simulink model "Geneva_Drive"  (R2015a)
settings: Solver=ode15s  StartTime=0.0  StopTime=30  MaxStep=1e-2  RelTol=1e-4  AbsTol=1e-5
PostLoadFcn:
  | set_param(bdroot,'IgnoredZcDiagnostic','none')
  | warning off sm:compiler:topologyAnalysis:DanglingBlock
StartFcn:
  | tic;
StopFcn:
  | Elapsed_Sim_Time = toc;
  | disp(['Elapsed Sim Time = ' num2str(Elapsed_Sim_Time)]);
undefined symbols (not defined in the file): X, Y, Z
libraries: sm_lib x44, Contact_Forces_Lib x20, nesl_utility x5, simulink x1
(part 1 of 2)
Description:
  | Copyright 2015 The MathWorks, Inc.
settings Model: CovSFcnEnable=off  Creator=smiller  LastModifiedBy=smiller
settings DataIOCC: LimitDataPoints=off  SaveFormat=StructureWithTime  SaveState=on
settings DebuggingCC: IgnoredZcDiagnostic=none  SolverPrmCheckMsg=warning
settings ExplorerConfigSet: InternalSimMechanicsExplorerSettings="<ExplorerConfiguration><canonicalview>default</canonicalview><AnimationSetting><BasePlaybackSpeed>1.0</BasePlaybackSpeed><PlaybackSpeedFactor>4.0</PlaybackSpeedFactor></AnimationSetting><TilePanel><TileInfo><Tiles Columns=\"1\" Count=\"1\" Rows=\"1\"><Column Left=\"2\" Weight=\"1\"/><Column Left=\"677\"/><Row Top=\"2\" Weight=\"1\"/><Row Top=\"558\"/><Tile Height=\"1\" Width=\"1\" X=\"0\" Y=\"0\"/></Tiles></TileInfo><SceneInfo><SceneViewer><BGColor><R>0.93725490570068359</R><G>0.9686274528503418</G><B>0.9686274528503418</B></BGColor><Camera><Position><X>0.26080521668652706</X><Y>0.4639017710068058</Y><Z>0.36701914488687676</Z></Position><Center><X>-0.034093618327655228</X><Y>0.025639318022065816</Y><Z>-0.010275526182887462</Z></Center><Up><X>-0.45579088703273962</X><Y>0.73671340761661774</Y><Z>-0.4995077800553458</Z></Up><Left>-0.33774445205926895</Left><Right>0.33774445205926895</Right><Bottom>-0.208832748234272</Bottom><Top>0.208832748234272</Top></Camera></SceneViewer></SceneInfo></TilePanel></ExplorerConfiguration>"

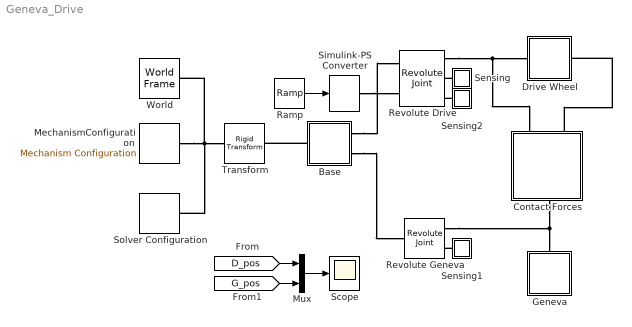
== system Geneva_Drive ==
  Base : Subsystem
  Contact Forces : Subsystem
  Drive Wheel : Subsystem
  Geneva : Subsystem
  MechanismConfiguration : sm_lib/Utilities/Mechanism Configuration  UniformGravity=Constant  GravityVector=[0 -9.81 0]  GravityUnits=m/s^2  LinearizationDelta=0.001  BlockFunction=simmechanics.library.utilities.mechanism_configuration
  Mux : Mux  Inputs=2
  Ramp : simulink/Sources/Ramp  slope=90  start=0  X0=106.26478005487978
  Revolute Drive : sm_lib/Joints/Revolute Joint  SenseConstraintForce=off  SenseConstraintForceX=off  SenseConstraintForceY=off  SenseConstraintForceZ=off  SenseConstraintTorque=off  SenseConstraintTorqueX=off  SenseConstraintTorqueY=off  SenseConstraintTorqueZ=off  SenseTotalForce=off  SenseTotalForceX=off  SenseTotalForceY=off  SenseTotalForceZ=off  SenseTotalTorque=off  SenseTotalTorqueX=off  SenseTotalTorqueY=off  SenseTotalTorqueZ=off  CompositeWrenchDir=FollowerOnBase  CompositeWrenchFrame=BaseFrame  EquilibriumPosition=0  EquilibriumPositionUnits=rad  SpringStiffness=0  SpringStiffnessUnits=m*N/rad  DampingCoefficient=0  DampingCoefficientUnits=m*s*N/rad  TorqueActuationMode=ComputedTorque  MotionActuationMode=InputMotion  SensePosition=on  SenseVelocity=off  SenseAcceleration=off  SenseTorqueForce=on  PositionTargetSpecify=on  PositionTargetPriority=Low  PositionTargetValue=106.26478005487978  PositionTargetValueUnits=deg  VelocityTargetSpecify=off  VelocityTargetPriority=High  VelocityTargetValue=0  VelocityTargetValueUnits=deg/s  BlockFunction=simmechanics.library.joints.revolute_joint
  Revolute Geneva : sm_lib/Joints/Revolute Joint  SenseConstraintForce=off  SenseConstraintForceX=off  SenseConstraintForceY=off  SenseConstraintForceZ=off  SenseConstraintTorque=off  SenseConstraintTorqueX=off  SenseConstraintTorqueY=off  SenseConstraintTorqueZ=off  SenseTotalForce=off  SenseTotalForceX=off  SenseTotalForceY=off  SenseTotalForceZ=off  SenseTotalTorque=off  SenseTotalTorqueX=off  SenseTotalTorqueY=off  SenseTotalTorqueZ=off  CompositeWrenchDir=FollowerOnBase  CompositeWrenchFrame=BaseFrame  EquilibriumPosition=90.000000000003197  EquilibriumPositionUnits=deg  SpringStiffness=0  SpringStiffnessUnits=m*N/rad  DampingCoefficient=1  DampingCoefficientUnits=m*s*N/rad  TorqueActuationMode=NoTorque  MotionActuationMode=ComputedMotion  SensePosition=on  SenseVelocity=off  SenseAcceleration=off  SenseTorqueForce=off  PositionTargetSpecify=on  PositionTargetPriority=Low  PositionTargetValue=90.000000000003197  PositionTargetValueUnits=deg  VelocityTargetSpecify=off  VelocityTargetPriority=High  VelocityTargetValue=0  VelocityTargetValueUnits=deg/s  BlockFunction=simmechanics.library.joints.revolute_joint
  Scope : Scope
      settings: YMin=0  YMax=8  SaveName=ScopeData3
  Sensing : Subsystem
  Sensing1 : Subsystem
  Sensing2 : Subsystem
  Simulink-PS Converter : nesl_utility/Simulink-PS Converter  PhysicalDomain=network_engine_domain  SubClassName=ps_input  LeftPortType=input  RightPortType=output  PseudoPeriodic=off  Frequencies=[]  NoiseDistribution=none  NoiseParameters=[]  Unit=deg  AffineConversion=off  InputFiltering=on  SimscapeFilterOrder=2  InputFilterTimeConstant=0.01  UdotUserProvided=1
  Solver Configuration : nesl_utility/Solver Configuration  PhysicalDomain=network_engine_domain  SubClassName=solver  LeftPortType=input  RightPortType=generic  Accelerate=off  Tones=[]  Harmonics=[]  SimulateNoise=off  Profile=off  UseLocalSampling=off  EnableSwitchedLinearOptims=on  FrequencyDomain=off  UseCCode=off  RelTol=0.001  AbsTol=1e-06  MinStep=1e-09  ToWorkspace=off  RevertToSquareIcSolve=off  NumHomotopyIterations=100  DoDC=off  ResidualTolerance=1e-09  UseLocalSolver=off  LocalSolverChoice=NE_BACKWARD_EULER_ADVANCER  LocalSolverSampleTime=0.001  DoFixedCost=off  MaxNonlinIter=3  MaxModeIter=2  LinearAlgebra=Sparse  DelaysMemoryBudget=1024  AutomaticFiltering=on  FilteringTimeConstant=0.001
  "Transform " : sm_lib/Frames and Transforms/Rigid Transform  TranslationMethod=Cartesian  TranslationLengthUnit=mm  TranslationStandardAxis=+Z  TranslationStandardOffset=0  TranslationCartesianOffset=[-30.994181557875464 40 -14.83110487348719]  TranslationROffset=0  TranslationROffsetUnits=m  TranslationZOffset=0  TranslationZOffsetUnits=m  TranslationThetaOffset=0  TranslationThetaOffsetUnits=deg  RotationMethod=ArbitraryAxis  RotationAngleUnits=rad  RotationStandardAxis=+Z  RotationAngle=1.5707963267948966  RotationArbitraryAxis=[-1 0 0]  FollAlignAxisA=+X  BaseAlignAxisA=+Y  FollAlignAxisB=+Y  BaseAlignAxisB=+Z  RotationMatrix=[1 0 0; 0 1 0; 0 0 1]  BlockFunction=simmechanics.library.frames_transforms.rigid_transform
  World : sm_lib/Frames and Transforms/World Frame  BlockFunction=simmechanics.library.frames_transforms.world_frame
  wires:
  Ramp/1 -> Simulink-PS Converter/1
  [D_pos] -> Mux/1
  Mux/1 -> Scope/1
  [G_pos] -> Mux/2
  connections:
  World/RConn1 -- "Transform "/LConn1 -- Solver Configuration/RConn1 -- MechanismConfiguration/RConn1
  Revolute Drive/RConn1 -- Drive Wheel/LConn1 -- Contact Forces/RConn1
  Revolute Geneva/RConn1 -- Geneva/LConn1 -- Contact Forces/LConn1
  Sensing2/LConn1 -- Revolute Drive/RConn3
  Sensing1/LConn1 -- Revolute Geneva/RConn2
  Sensing/LConn1 -- Revolute Drive/RConn2
  Contact Forces/RConn2 -- Drive Wheel/RConn1
  Simulink-PS Converter/RConn1 -- Revolute Drive/LConn2
  Base/LConn1 -- "Transform "/RConn1
  Base/RConn1 -- Revolute Drive/LConn1
  Base/RConn2 -- Revolute Geneva/LConn1

== system Geneva_Drive/Base ==
  ReferenceFrame : sm_lib/Frames and Transforms/Reference Frame  BlockFunction=simmechanics.library.frames_transforms.reference_frame
  Solid : sm_lib/Body Elements/Solid  InertiaType=Custom  Mass=5.6121441650895836  MassUnits=kg  CenterOfMass=[0.22415415704528135 0 -24.782168314450626]  CenterOfMassUnits=mm  MomentsOfInertia=[57246.923822174664 131168.16755878026 187513.90774897448]  MomentsOfInertiaUnits=kg*mm^2  ProductsOfInertia=[0 -24.879239071091789 0]  ProductsOfInertiaUnits=kg*mm^2  DensityBased=on  Density=1000  DensityUnits=kg/(m^3)  GraphicType=FromGeometry  MarkerShape=Sphere  MarkerSize=10  MarkerSizeUnits=m  GraphicVisPropType=SimpleVisualProperties  GraphicDiffuseColor=[0.82745098039215681 0.82745098039215681 0.81960784313725488]  GraphicSpecularColor=[0.5 0.5 0.5 1.0]  GraphicAmbientColor=[0.15 0.15 0.15 1.0]  GraphicEmissiveColor=[0.0 0.0 0.0 1.0]  GraphicShininess=75  GraphicOpacity=1  GeometryShape=FromFile  RectangleSize=[1 1]  RectangleSizeUnits=m  BrickDimensions=[1 1 1]  BrickDimensionUnits=m  CylinderRadius=1  CylinderRadiusUnits=m  CylinderLength=1  CylinderLengthUnits=m  SphereRadius=1  SphereRadiusUnits=m  EllipsoidRadii=[1 1 1]  EllipsoidRadiiUnits=m  ExtrusionCrossSection=[1 1; -1 1; -1 -1; 1 -1]  ExtrusionCrossSectionUnits=m  ExtrusionLength=1  ExtrusionLengthUnits=m  PolygonNumSides=3  PolygonOuterRadius=1  PolygonOuterRadiusUnits=m  ExtGeomFileType=STL  ExtGeomFileName=Base_Default_sldprt.STL  ExtGeomFileUnits=mm  RevolutionCrossSection=[1 1; 1 -1; 2 -1; 2 1]  RevolutionCrossSectionUnits=m  RevolutionExtent=Full  RevolutionAngle=180  RevolutionAngleUnits=deg  BlockFunction=simmechanics.library.body_elements.solid
  Transform : sm_lib/Frames and Transforms/Rigid Transform  TranslationMethod=Cartesian  TranslationLengthUnit=mm  TranslationStandardAxis=+Z  TranslationStandardOffset=0  TranslationCartesianOffset=[100 0 0]  TranslationROffset=0  TranslationROffsetUnits=m  TranslationZOffset=0  TranslationZOffsetUnits=m  TranslationThetaOffset=0  TranslationThetaOffsetUnits=deg  RotationMethod=ArbitraryAxis  RotationAngleUnits=rad  RotationStandardAxis=+Z  RotationAngle=0  RotationArbitraryAxis=[0 0 0]  FollAlignAxisA=+X  BaseAlignAxisA=+Y  FollAlignAxisB=+Y  BaseAlignAxisB=+Z  RotationMatrix=[1 0 0; 0 1 0; 0 0 1]  BlockFunction=simmechanics.library.frames_transforms.rigid_transform
  Transform2 : sm_lib/Frames and Transforms/Rigid Transform  TranslationMethod=Cartesian  TranslationLengthUnit=mm  TranslationStandardAxis=+Z  TranslationStandardOffset=0  TranslationCartesianOffset=[-99.999999999999986 0 57.42640687119286]  TranslationROffset=0  TranslationROffsetUnits=m  TranslationZOffset=0  TranslationZOffsetUnits=m  TranslationThetaOffset=0  TranslationThetaOffsetUnits=deg  RotationMethod=ArbitraryAxis  RotationAngleUnits=rad  RotationStandardAxis=+Z  RotationAngle=3.1415926535897931  RotationArbitraryAxis=[1 0 0]  FollAlignAxisA=+X  BaseAlignAxisA=+Y  FollAlignAxisB=+Y  BaseAlignAxisB=+Z  RotationMatrix=[1 0 0; 0 1 0; 0 0 1]  BlockFunction=simmechanics.library.frames_transforms.rigid_transform
  F3 : PMIOPort  Port=1  Side=Left
  F2 : PMIOPort  Port=2  Side=Right
  F : PMIOPort  Port=3  Side=Right
  connections:
  Transform2/RConn1 -- F2/RConn1
  Transform/RConn1 -- F/RConn1
  F3/RConn1 -- Transform2/LConn1 -- Transform/LConn1 -- ReferenceFrame/RConn1 -- Solid/RConn1

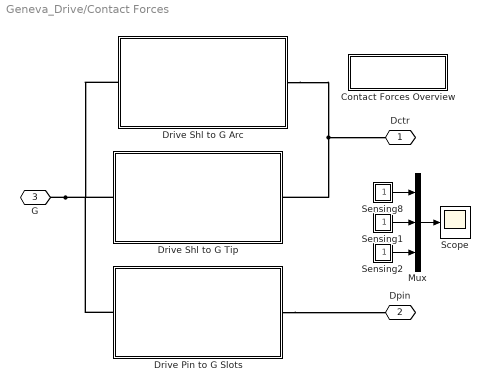
== system Geneva_Drive/Contact Forces ==
  Contact Forces Overview : Subsystem
      settings: OpenFcn=web(which('Geneva_Drive_Contact_Forces.html'));
      mask Display: disp('Contact Forces\nOverview');
  Drive Pin to G Slots : Subsystem  mask(Contact Forces, Drive Pin and Geneva Slot){k_contact=1e5, b_contact=1e4, r_drive_pin=0.015, d_genv_lin=0.0055, l_genv_lin=0.1405*2}
      mask prompts: k_contact "Contact Stiffness (N/m)"; b_contact "Contact Damping (N/(m/s))"; r_drive_pin "Radius of Drive Wheel Pin (m)"; d_genv_lin "Line Thickness, Geneva Slot Contact (m)"; l_genv_lin "Slot Length Through Geneva (m)"
      mask help:
      | This subsystem models the contact forces between the drive wheel pin and the four slots on the Geneva.  All contact forces are identical.  They connect one reference frame on the drive wheel pin and four reference frames on the Geneva.
      |
      | Click the Help button for a diagram of the contact forces and the parameters.
      mask Help: web(which('Geneva_Drive_Contact_DPin_GSlot.html'));
      mask Display:
      | image(imread('Contact_Diagram_Dpin_to_GSlot_IMAGE.jpg'));
      | port_label('LConn',1,'LinB');
      | port_label('RConn',1,'CirF');
  Drive Shl to G Arc : Subsystem  mask(Contact Forces, Drive Shoulder and Geneva Arc){k_contact=1e4, b_contact=1e2, r_shld_cir=0.005, r_genv_xcir=0.115, d_genv_xcir=0.005, d_genv_ctr_to_xcir=0.2}
      mask prompts: k_contact "Contact Stiffness (N/m)"; b_contact "Contact Damping (N/(m/s))"; r_shld_cir "Circle Radius of Drive Wheel Shoulder Contact (m)"; r_genv_xcir "Ring Radius, Geneva Arc (m)"; d_genv_xcir "Ring Thickness, Geneva Arc Contact (m)"; d_genv_ctr_to_xcir "Distance Geneva axis to center exterior circle (m)"
      mask help:
      | This subsystem models the contact forces between the drive wheel shoulder and the exterior arcs on the Geneva.  All contact forces are identical.  They connect two reference frames on the drive wheel and four reference frames on the Geneva.
      |
      | Click the Help button for a diagram of the contact forces and the parameters.
      mask Help: web(which('Geneva_Drive_Contact_Shld_Garc.html'));
      mask Display:
      | image(imread('Contact_Diagram_Shld_to_GArc_IMAGE.jpg'));
      | port_label('Lconn',1,'RinB');
      | port_label('Rconn',1,'CirF');
  Drive Shl to G Tip : Subsystem  mask(Contact Forces, Drive Shoulder and Geneva Tips){k_contact=1e4, b_contact=1e2, r_genv_cir=0.0045, r_shld=0.115, d_shld=0.005}
      mask prompts: k_contact "Contact Stiffness (N/m)"; b_contact "Contact Damping (N/(m/s))"; r_genv_cir "Circle Radius, Geneva Tip Contact (m)"; r_shld "Ring Radius, Drive Wheel Shoulder (m)"; d_shld "Ring Thickness, Drive Wheel Shoulder Contact (m)"
      mask help:
      | This subsystem models the contact forces between the drive wheel shoulder and the tips of the Geneva.  All contact forces are identical.  They connect one reference frame on the drive wheel and eight reference frames on the Geneva.
      |
      | Click the Help button for a diagram of the contact forces and the parameters.
      mask Help: web(which('Geneva_Drive_Contact_Shld_Gtip.html'));
      mask Display:
      | image(imread('Contact_Diagram_Gtip_to_Shld_IMAGE.jpg'));
      | port_label('Lconn',1,'CirF');
      | port_label('Rconn',1,'RinB');
  Mux : Mux  Inputs=3
  Scope : Scope
      settings: YMin=-10  YMax=60  SaveName=ScopeData5
  Sensing1 : Subsystem
  Sensing2 : Subsystem
  Sensing8 : Subsystem
  Dctr : PMIOPort  Port=1  Side=Right
  Dpin : PMIOPort  Port=2  Side=Right
  G : PMIOPort  Port=3  Side=Left
  wires:
  Mux/1 -> Scope/1
  Sensing2/1(S) -> Mux/3
  Sensing1/1(S) -> Mux/2
  Sensing8/1(S) -> Mux/1
  connections:
  G/RConn1 -- Drive Shl to G Arc/LConn1 -- Drive Pin to G Slots/LConn1 -- Drive Shl to G Tip/LConn1
  Drive Pin to G Slots/RConn1 -- Dpin/RConn1
  Drive Shl to G Arc/RConn1 -- Dctr/RConn1 -- Drive Shl to G Tip/RConn1

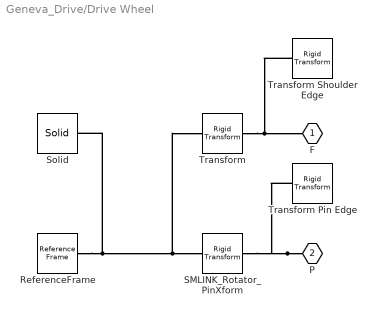
== system Geneva_Drive/Drive Wheel ==
  ReferenceFrame : sm_lib/Frames and Transforms/Reference Frame  BlockFunction=simmechanics.library.frames_transforms.reference_frame
  SMLINK_Rotator_PinXform : sm_lib/Frames and Transforms/Rigid Transform  TranslationMethod=Cartesian  TranslationLengthUnit=mm  TranslationStandardAxis=+Z  TranslationStandardOffset=0  TranslationCartesianOffset=[0 99.999999999999943 1.0000000000000009]  TranslationROffset=0  TranslationROffsetUnits=m  TranslationZOffset=0  TranslationZOffsetUnits=m  TranslationThetaOffset=0  TranslationThetaOffsetUnits=deg  RotationMethod=StandardAxis  RotationAngleUnits=deg  RotationStandardAxis=+Z  RotationAngle=10  RotationArbitraryAxis=[0 0 1]  FollAlignAxisA=+X  BaseAlignAxisA=+Y  FollAlignAxisB=+Y  BaseAlignAxisB=+Z  RotationMatrix=[1 0 0; 0 1 0; 0 0 1]  BlockFunction=simmechanics.library.frames_transforms.rigid_transform
  Solid : sm_lib/Body Elements/Solid  InertiaType=Custom  Mass=1.1459440199505517  MassUnits=kg  CenterOfMass=[-103.32572655678197 -3.3257265567819814 0.56035000006051983]  CenterOfMassUnits=mm  MomentsOfInertia=[5063.1142307875289 5063.1142307875298 10008.151794093599]  MomentsOfInertiaUnits=kg*mm^2  ProductsOfInertia=[46.956086417341879 46.956086417341901 41.94861289102812]  ProductsOfInertiaUnits=kg*mm^2  DensityBased=on  Density=1000  DensityUnits=kg/(m^3)  GraphicType=FromGeometry  MarkerShape=Sphere  MarkerSize=10  MarkerSizeUnits=m  GraphicVisPropType=SimpleVisualProperties  GraphicDiffuseColor=[0.2 0.4 1.0]  GraphicSpecularColor=[0.5 0.5 0.5 1.0]  GraphicAmbientColor=[0.15 0.15 0.15 1.0]  GraphicEmissiveColor=[0.0 0.0 0.0 1.0]  GraphicShininess=75  GraphicOpacity=1  GeometryShape=FromFile  RectangleSize=[1 1]  RectangleSizeUnits=m  BrickDimensions=[1 1 1]  BrickDimensionUnits=m  CylinderRadius=1  CylinderRadiusUnits=m  CylinderLength=1  CylinderLengthUnits=m  SphereRadius=1  SphereRadiusUnits=m  EllipsoidRadii=[1 1 1]  EllipsoidRadiiUnits=m  ExtrusionCrossSection=[1 1; -1 1; -1 -1; 1 -1]  ExtrusionCrossSectionUnits=m  ExtrusionLength=1  ExtrusionLengthUnits=m  PolygonNumSides=3  PolygonOuterRadius=1  PolygonOuterRadiusUnits=m  ExtGeomFileType=STL  ExtGeomFileName=Drive_Wheel_Default_sldprt.STL  ExtGeomFileUnits=mm  RevolutionCrossSection=[1 1; 1 -1; 2 -1; 2 1]  RevolutionCrossSectionUnits=m  RevolutionExtent=Full  RevolutionAngle=180  RevolutionAngleUnits=deg  BlockFunction=simmechanics.library.body_elements.solid
  Transform : sm_lib/Frames and Transforms/Rigid Transform  TranslationMethod=Cartesian  TranslationLengthUnit=mm  TranslationStandardAxis=+Z  TranslationStandardOffset=0  TranslationCartesianOffset=[-100.00000000000026 2.1316282072803006e-14 57.426406871192782]  TranslationROffset=0  TranslationROffsetUnits=m  TranslationZOffset=0  TranslationZOffsetUnits=m  TranslationThetaOffset=0  TranslationThetaOffsetUnits=deg  RotationMethod=ArbitraryAxis  RotationAngleUnits=rad  RotationStandardAxis=+Z  RotationAngle=3.1415926535897931  RotationArbitraryAxis=[-1 5.9163189700902024e-33 -6.6609835156154749e-17]  FollAlignAxisA=+X  BaseAlignAxisA=+Y  FollAlignAxisB=+Y  BaseAlignAxisB=+Z  RotationMatrix=[1 0 0; 0 1 0; 0 0 1]  BlockFunction=simmechanics.library.frames_transforms.rigid_transform
  Transform Pin Edge : sm_lib/Frames and Transforms/Rigid Transform  TranslationMethod=StandardAxis  TranslationLengthUnit=m  TranslationStandardAxis=+X  TranslationStandardOffset=0.015  TranslationCartesianOffset=[0 0 0]  TranslationROffset=0.115  TranslationROffsetUnits=m  TranslationZOffset=0  TranslationZOffsetUnits=m  TranslationThetaOffset=270  TranslationThetaOffsetUnits=deg  RotationMethod=None  RotationAngleUnits=deg  RotationStandardAxis=+Z  RotationAngle=0  RotationArbitraryAxis=[0 0 1]  FollAlignAxisA=+X  BaseAlignAxisA=+Y  FollAlignAxisB=+Y  BaseAlignAxisB=+Z  RotationMatrix=[1 0 0; 0 1 0; 0 0 1]  BlockFunction=simmechanics.library.frames_transforms.rigid_transform
  Transform Shoulder Edge : sm_lib/Frames and Transforms/Rigid Transform  TranslationMethod=Cylindrical  TranslationLengthUnit=m  TranslationStandardAxis=+X  TranslationStandardOffset=0.115  TranslationCartesianOffset=[0 0 0]  TranslationROffset=0.115  TranslationROffsetUnits=m  TranslationZOffset=0  TranslationZOffsetUnits=m  TranslationThetaOffset=270  TranslationThetaOffsetUnits=deg  RotationMethod=None  RotationAngleUnits=deg  RotationStandardAxis=+Z  RotationAngle=0  RotationArbitraryAxis=[0 0 1]  FollAlignAxisA=+X  BaseAlignAxisA=+Y  FollAlignAxisB=+Y  BaseAlignAxisB=+Z  RotationMatrix=[1 0 0; 0 1 0; 0 0 1]  BlockFunction=simmechanics.library.frames_transforms.rigid_transform
  F : PMIOPort  Port=1  Side=Left
  P : PMIOPort  Port=2  Side=Right
  connections:
  Transform Shoulder Edge/LConn1 -- F/RConn1 -- Transform/RConn1
  P/RConn1 -- Transform Pin Edge/LConn1 -- SMLINK_Rotator_PinXform/RConn1
  ReferenceFrame/RConn1 -- Solid/RConn1 -- Transform/LConn1 -- SMLINK_Rotator_PinXform/LConn1

== system Geneva_Drive/Geneva ==
  ReferenceFrame : sm_lib/Frames and Transforms/Reference Frame  BlockFunction=simmechanics.library.frames_transforms.reference_frame
  Solid : sm_lib/Body Elements/Solid  InertiaType=Custom  Mass=0.24105441419713447  MassUnits=kg  CenterOfMass=[100.00000000000023 1.1564451014440063e-12 5.0000000000000009]  CenterOfMassUnits=mm  MomentsOfInertia=[803.62795532691052 803.62795532691234 1603.261580672231]  MomentsOfInertiaUnits=kg*mm^2  ProductsOfInertia=[0 0 0]  ProductsOfInertiaUnits=kg*mm^2  DensityBased=on  Density=1000  DensityUnits=kg/(m^3)  GraphicType=FromGeometry  MarkerShape=Sphere  MarkerSize=10  MarkerSizeUnits=m  GraphicVisPropType=SimpleVisualProperties  GraphicDiffuseColor=[1.0 0.4 0.0]  GraphicSpecularColor=[0.5 0.5 0.5 1.0]  GraphicAmbientColor=[0.15 0.15 0.15 1.0]  GraphicEmissiveColor=[0.0 0.0 0.0 1.0]  GraphicShininess=75  GraphicOpacity=1  GeometryShape=FromFile  RectangleSize=[1 1]  RectangleSizeUnits=m  BrickDimensions=[1 1 1]  BrickDimensionUnits=m  CylinderRadius=1  CylinderRadiusUnits=m  CylinderLength=1  CylinderLengthUnits=m  SphereRadius=1  SphereRadiusUnits=m  EllipsoidRadii=[1 1 1]  EllipsoidRadiiUnits=m  ExtrusionCrossSection=[1 1; -1 1; -1 -1; 1 -1]  ExtrusionCrossSectionUnits=m  ExtrusionLength=1  ExtrusionLengthUnits=m  PolygonNumSides=3  PolygonOuterRadius=1  PolygonOuterRadiusUnits=m  ExtGeomFileType=STL  ExtGeomFileName=Geneva_Default_sldprt.STL  ExtGeomFileUnits=mm  RevolutionCrossSection=[1 1; 1 -1; 2 -1; 2 1]  RevolutionCrossSectionUnits=m  RevolutionExtent=Full  RevolutionAngle=180  RevolutionAngleUnits=deg  BlockFunction=simmechanics.library.body_elements.solid
  Transform Ref to Ctr : sm_lib/Frames and Transforms/Rigid Transform  TranslationMethod=Cartesian  TranslationLengthUnit=mm  TranslationStandardAxis=+Z  TranslationStandardOffset=0  TranslationCartesianOffset=[99.999999999999261 -2.4158453015843406e-13 -1.4210854715202004e-14]  TranslationROffset=0  TranslationROffsetUnits=m  TranslationZOffset=0  TranslationZOffsetUnits=m  TranslationThetaOffset=0  TranslationThetaOffsetUnits=deg  RotationMethod=ArbitraryAxis  RotationAngleUnits=rad  RotationStandardAxis=+Z  RotationAngle=0  RotationArbitraryAxis=[0 0 0]  FollAlignAxisA=+X  BaseAlignAxisA=+Y  FollAlignAxisB=+Y  BaseAlignAxisB=+Z  RotationMatrix=[1 0 0; 0 1 0; 0 0 1]  BlockFunction=simmechanics.library.frames_transforms.rigid_transform
  F : PMIOPort  Port=1  Side=Left
  connections:
  F/RConn1 -- Transform Ref to Ctr/RConn1
  Transform Ref to Ctr/LConn1 -- ReferenceFrame/RConn1 -- Solid/RConn1

== system Geneva_Drive/Sensing ==
  PS-Simulink Converter : nesl_utility/PS-Simulink Converter  PhysicalDomain=network_engine_domain  SubClassName=ps_output  LeftPortType=input  RightPortType=output  PseudoPeriodic=off  Frequencies=[]  Unit=rev  AffineConversion=off
  S : PMIOPort  Port=1  Side=Left
  tag scope: D_pos=global
  wires:
  PS-Simulink Converter/1 -> [D_pos]
  connections:
  PS-Simulink Converter/LConn1 -- S/RConn1

== system Geneva_Drive/Sensing1 ==
  PS-Simulink Converter : nesl_utility/PS-Simulink Converter  PhysicalDomain=network_engine_domain  SubClassName=ps_output  LeftPortType=input  RightPortType=output  PseudoPeriodic=off  Frequencies=[]  Unit=rev  AffineConversion=off
  S : PMIOPort  Port=1  Side=Left
  tag scope: G_pos=global
  wires:
  PS-Simulink Converter/1 -> [G_pos]
  connections:
  PS-Simulink Converter/LConn1 -- S/RConn1

== system Geneva_Drive/Sensing2 ==
  PS-Simulink Converter : nesl_utility/PS-Simulink Converter  PhysicalDomain=network_engine_domain  SubClassName=ps_output  LeftPortType=input  RightPortType=output  PseudoPeriodic=off  Frequencies=[]  Unit=1  AffineConversion=off
  Scope : Scope
  S : PMIOPort  Port=1  Side=Left
  wires:
  PS-Simulink Converter/1 -> Scope/1
  connections:
  PS-Simulink Converter/LConn1 -- S/RConn1

== system Geneva_Drive/Contact Forces/Contact Forces Overview ==

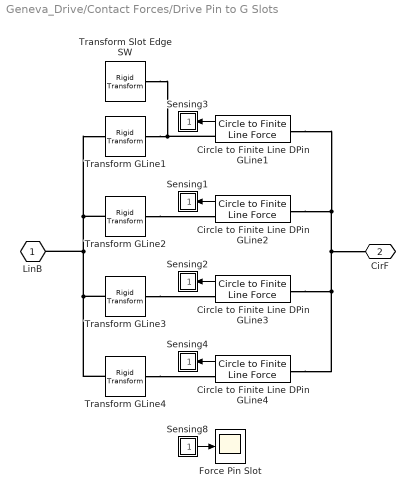
== system Geneva_Drive/Contact Forces/Drive Pin to G Slots ==
  Circle to Finite Line DPin GLine{1..4} (4 alike) : Contact_Forces_Lib/2D/Circle to Finite Line Force  circle_rad=r_drive_pin  line_depth=d_genv_lin  line_length=l_genv_lin  force_law=Linear  k_contact=k_contact  b_contact=b_contact  pen_full_damp_F=1e-4  pen_exponent=1  custom_param_1=1  custom_param_2=1  friction_law=None  mu_kinetic=0.5  mu_static=0.7  v_thr=0.001
  Force Pin Slot : Scope
      settings: YMin=0  YMax=60
  Sensing1 : Subsystem
  Sensing2 : Subsystem
  Sensing3 : Subsystem
  Sensing4 : Subsystem
  Sensing8 : Subsystem
  Transform GLine1 : sm_lib/Frames and Transforms/Rigid Transform  TranslationMethod=Cylindrical  TranslationLengthUnit=m  TranslationStandardAxis=+Z  TranslationStandardOffset=0  TranslationCartesianOffset=[0 0 0]  TranslationROffset=-0.02  TranslationROffsetUnits=m  TranslationZOffset=0  TranslationZOffsetUnits=m  TranslationThetaOffset=315  TranslationThetaOffsetUnits=deg  RotationMethod=StandardAxis  RotationAngleUnits=deg  RotationStandardAxis=+Z  RotationAngle=315  RotationArbitraryAxis=[0 0 1]  FollAlignAxisA=+X  BaseAlignAxisA=+Y  FollAlignAxisB=+Y  BaseAlignAxisB=+Z  RotationMatrix=[1 0 0; 0 1 0; 0 0 1]  BlockFunction=simmechanics.library.frames_transforms.rigid_transform
  Transform GLine2 : sm_lib/Frames and Transforms/Rigid Transform  TranslationMethod=Cylindrical  TranslationLengthUnit=m  TranslationStandardAxis=+Z  TranslationStandardOffset=0  TranslationCartesianOffset=[0 0 0]  TranslationROffset=-0.02  TranslationROffsetUnits=m  TranslationZOffset=0  TranslationZOffsetUnits=m  TranslationThetaOffset=135  TranslationThetaOffsetUnits=deg  RotationMethod=StandardAxis  RotationAngleUnits=deg  RotationStandardAxis=+Z  RotationAngle=135  RotationArbitraryAxis=[0 0 1]  FollAlignAxisA=+X  BaseAlignAxisA=+Y  FollAlignAxisB=+Y  BaseAlignAxisB=+Z  RotationMatrix=[1 0 0; 0 1 0; 0 0 1]  BlockFunction=simmechanics.library.frames_transforms.rigid_transform
  Transform GLine3 : sm_lib/Frames and Transforms/Rigid Transform  TranslationMethod=Cylindrical  TranslationLengthUnit=m  TranslationStandardAxis=+Z  TranslationStandardOffset=0  TranslationCartesianOffset=[0 0 0]  TranslationROffset=-0.02  TranslationROffsetUnits=m  TranslationZOffset=0  TranslationZOffsetUnits=m  TranslationThetaOffset=225  TranslationThetaOffsetUnits=deg  RotationMethod=StandardAxis  RotationAngleUnits=deg  RotationStandardAxis=+Z  RotationAngle=225  RotationArbitraryAxis=[0 0 1]  FollAlignAxisA=+X  BaseAlignAxisA=+Y  FollAlignAxisB=+Y  BaseAlignAxisB=+Z  RotationMatrix=[1 0 0; 0 1 0; 0 0 1]  BlockFunction=simmechanics.library.frames_transforms.rigid_transform
  Transform GLine4 : sm_lib/Frames and Transforms/Rigid Transform  TranslationMethod=Cylindrical  TranslationLengthUnit=m  TranslationStandardAxis=+Z  TranslationStandardOffset=0  TranslationCartesianOffset=[0 0 0]  TranslationROffset=-0.02  TranslationROffsetUnits=m  TranslationZOffset=0  TranslationZOffsetUnits=m  TranslationThetaOffset=45  TranslationThetaOffsetUnits=deg  RotationMethod=StandardAxis  RotationAngleUnits=deg  RotationStandardAxis=+Z  RotationAngle=45  RotationArbitraryAxis=[0 0 1]  FollAlignAxisA=+X  BaseAlignAxisA=+Y  FollAlignAxisB=+Y  BaseAlignAxisB=+Z  RotationMatrix=[1 0 0; 0 1 0; 0 0 1]  BlockFunction=simmechanics.library.frames_transforms.rigid_transform
  Transform Slot Edge SW : sm_lib/Frames and Transforms/Rigid Transform  TranslationMethod=StandardAxis  TranslationLengthUnit=m  TranslationStandardAxis=+X  TranslationStandardOffset=0.005  TranslationCartesianOffset=[0 0 0]  TranslationROffset=0  TranslationROffsetUnits=m  TranslationZOffset=0  TranslationZOffsetUnits=m  TranslationThetaOffset=0  TranslationThetaOffsetUnits=deg  RotationMethod=None  RotationAngleUnits=deg  RotationStandardAxis=+Z  RotationAngle=45  RotationArbitraryAxis=[0 0 1]  FollAlignAxisA=+X  BaseAlignAxisA=+Y  FollAlignAxisB=+Y  BaseAlignAxisB=+Z  RotationMatrix=[1 0 0; 0 1 0; 0 0 1]  BlockFunction=simmechanics.library.frames_transforms.rigid_transform
  LinB : PMIOPort  Port=1  Side=Left
  CirF : PMIOPort  Port=2  Side=Right
  wires:
  Sensing8/1(S) -> Force Pin Slot/1
  Circle to Finite Line DPin GLine4/1 -> Sensing4/1(S)
  Circle to Finite Line DPin GLine3/1 -> Sensing2/1(S)
  Circle to Finite Line DPin GLine2/1 -> Sensing1/1(S)
  Circle to Finite Line DPin GLine1/1 -> Sensing3/1(S)
  connections:
  Transform GLine2/RConn1 -- Circle to Finite Line DPin GLine2/RConn1
  Transform GLine3/RConn1 -- Circle to Finite Line DPin GLine3/RConn1
  Circle to Finite Line DPin GLine4/LConn1 -- CirF/RConn1 -- Circle to Finite Line DPin GLine2/LConn1 -- Circle to Finite Line DPin GLine1/LConn1 -- Circle to Finite Line DPin GLine3/LConn1
  Transform Slot Edge SW/LConn1 -- Transform GLine1/RConn1 -- Circle to Finite Line DPin GLine1/RConn1
  Transform GLine4/RConn1 -- Circle to Finite Line DPin GLine4/RConn1
  Transform GLine3/LConn1 -- LinB/RConn1 -- Transform GLine2/LConn1 -- Transform GLine1/LConn1 -- Transform GLine4/LConn1

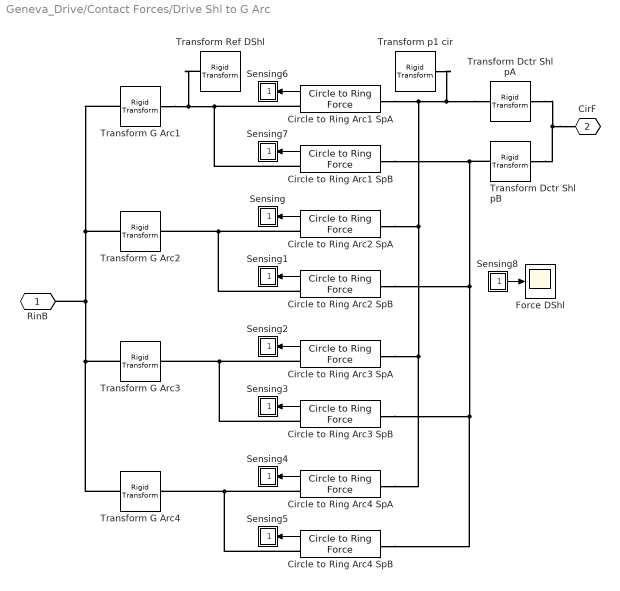
== system Geneva_Drive/Contact Forces/Drive Shl to G Arc ==
  "Circle to Ring Arc1 SpA " : Contact_Forces_Lib/2D/Circle to Ring Force  radius_circle=r_shld_cir  radius_ring=r_genv_xcir+d_genv_xcir/2  d_ring=d_genv_xcir  active_angle=[-45 45]  force_law=Linear  k_contact=k_contact  b_contact=b_contact  pen_full_damp_F=1e-4  pen_exponent=1  custom_param_1=1  custom_param_2=1  friction_law=None  mu_kinetic=0.5  mu_static=0.7  v_thr=0.001
  Circle to Ring Arc1 SpB : Contact_Forces_Lib/2D/Circle to Ring Force  radius_circle=r_shld_cir  radius_ring=r_genv_xcir+d_genv_xcir/2  d_ring=d_genv_xcir  active_angle=[-45 45]  force_law=Linear  k_contact=k_contact  b_contact=b_contact  pen_full_damp_F=1e-4  pen_exponent=1  custom_param_1=1  custom_param_2=1  friction_law=None  mu_kinetic=0.5  mu_static=0.7  v_thr=0.001
  Circle to Ring Arc2 SpA : Contact_Forces_Lib/2D/Circle to Ring Force  radius_circle=r_shld_cir  radius_ring=r_genv_xcir+d_genv_xcir/2  d_ring=d_genv_xcir  active_angle=[-45 45]  force_law=Linear  k_contact=k_contact  b_contact=b_contact  pen_full_damp_F=1e-4  pen_exponent=1  custom_param_1=1  custom_param_2=1  friction_law=None  mu_kinetic=0.5  mu_static=0.7  v_thr=0.001
  Circle to Ring Arc2 SpB : Contact_Forces_Lib/2D/Circle to Ring Force  radius_circle=r_shld_cir  radius_ring=r_genv_xcir+d_genv_xcir/2  d_ring=d_genv_xcir  active_angle=[-45 45]  force_law=Linear  k_contact=k_contact  b_contact=b_contact  pen_full_damp_F=1e-4  pen_exponent=1  custom_param_1=1  custom_param_2=1  friction_law=None  mu_kinetic=0.5  mu_static=0.7  v_thr=0.001
  Circle to Ring Arc3 SpA : Contact_Forces_Lib/2D/Circle to Ring Force  radius_circle=r_shld_cir  radius_ring=r_genv_xcir+d_genv_xcir/2  d_ring=d_genv_xcir  active_angle=[-45 45]  force_law=Linear  k_contact=k_contact  b_contact=b_contact  pen_full_damp_F=1e-4  pen_exponent=1  custom_param_1=1  custom_param_2=1  friction_law=None  mu_kinetic=0.5  mu_static=0.7  v_thr=0.001
  Circle to Ring Arc3 SpB : Contact_Forces_Lib/2D/Circle to Ring Force  radius_circle=r_shld_cir  radius_ring=r_genv_xcir+d_genv_xcir/2  d_ring=d_genv_xcir  active_angle=[-45 45]  force_law=Linear  k_contact=k_contact  b_contact=b_contact  pen_full_damp_F=1e-4  pen_exponent=1  custom_param_1=1  custom_param_2=1  friction_law=None  mu_kinetic=0.5  mu_static=0.7  v_thr=0.001
  Circle to Ring Arc4 SpA : Contact_Forces_Lib/2D/Circle to Ring Force  radius_circle=r_shld_cir  radius_ring=r_genv_xcir+d_genv_xcir/2  d_ring=d_genv_xcir  active_angle=[-45 45]  force_law=Linear  k_contact=k_contact  b_contact=b_contact  pen_full_damp_F=1e-4  pen_exponent=1  custom_param_1=1  custom_param_2=1  friction_law=None  mu_kinetic=0.5  mu_static=0.7  v_thr=0.001
  Circle to Ring Arc4 SpB : Contact_Forces_Lib/2D/Circle to Ring Force  radius_circle=r_shld_cir  radius_ring=r_genv_xcir+d_genv_xcir/2  d_ring=d_genv_xcir  active_angle=[-45 45]  force_law=Linear  k_contact=k_contact  b_contact=b_contact  pen_full_damp_F=1e-4  pen_exponent=1  custom_param_1=1  custom_param_2=1  friction_law=None  mu_kinetic=0.5  mu_static=0.7  v_thr=0.001
  Force DShl : Scope
      settings: TimeRange=30  YMin=-25  YMax=0  SaveName=ScopeData4
  Sensing : Subsystem
  Sensing1 : Subsystem
  Sensing2 : Subsystem
  Sensing3 : Subsystem
  Sensing4 : Subsystem
  Sensing5 : Subsystem
  Sensing6 : Subsystem
  Sensing7 : Subsystem
  Sensing8 : Subsystem
  Transform Dctr Shl pA : sm_lib/Frames and Transforms/Rigid Transform  TranslationMethod=StandardAxis  TranslationLengthUnit=m  TranslationStandardAxis=+X  TranslationStandardOffset=r_genv_xcir-r_shld_cir  TranslationCartesianOffset=[0 0 0]  TranslationROffset=0  TranslationROffsetUnits=m  TranslationZOffset=0  TranslationZOffsetUnits=m  TranslationThetaOffset=0  TranslationThetaOffsetUnits=deg  RotationMethod=None  RotationAngleUnits=deg  RotationStandardAxis=+X  RotationAngle=180  RotationArbitraryAxis=[0 0 1]  FollAlignAxisA=+X  BaseAlignAxisA=+Y  FollAlignAxisB=+Y  BaseAlignAxisB=+Z  RotationMatrix=[1 0 0; 0 1 0; 0 0 1]  BlockFunction=simmechanics.library.frames_transforms.rigid_transform
  Transform Dctr Shl pB : sm_lib/Frames and Transforms/Rigid Transform  TranslationMethod=StandardAxis  TranslationLengthUnit=m  TranslationStandardAxis=-Y  TranslationStandardOffset=r_genv_xcir-r_shld_cir  TranslationCartesianOffset=[0 0 0]  TranslationROffset=0  TranslationROffsetUnits=m  TranslationZOffset=0  TranslationZOffsetUnits=m  TranslationThetaOffset=0  TranslationThetaOffsetUnits=deg  RotationMethod=None  RotationAngleUnits=deg  RotationStandardAxis=+Z  RotationAngle=180  RotationArbitraryAxis=[0 0 1]  FollAlignAxisA=+X  BaseAlignAxisA=+Y  FollAlignAxisB=+Y  BaseAlignAxisB=+Z  RotationMatrix=[1 0 0; 0 1 0; 0 0 1]  BlockFunction=simmechanics.library.frames_transforms.rigid_transform
  Transform G Arc1 : sm_lib/Frames and Transforms/Rigid Transform  TranslationMethod=StandardAxis  TranslationLengthUnit=m  TranslationStandardAxis=+Y  TranslationStandardOffset=d_genv_ctr_to_xcir  TranslationCartesianOffset=[0 0 0]  TranslationROffset=0  TranslationROffsetUnits=m  TranslationZOffset=0  TranslationZOffsetUnits=m  TranslationThetaOffset=0  TranslationThetaOffsetUnits=deg  RotationMethod=StandardAxis  RotationAngleUnits=deg  RotationStandardAxis=+Z  RotationAngle=-90  RotationArbitraryAxis=[0 0 1]  FollAlignAxisA=+X  BaseAlignAxisA=+Y  FollAlignAxisB=+Y  BaseAlignAxisB=+Z  RotationMatrix=[1 0 0; 0 1 0; 0 0 1]  BlockFunction=simmechanics.library.frames_transforms.rigid_transform
  Transform G Arc2 : sm_lib/Frames and Transforms/Rigid Transform  TranslationMethod=StandardAxis  TranslationLengthUnit=m  TranslationStandardAxis=+X  TranslationStandardOffset=d_genv_ctr_to_xcir  TranslationCartesianOffset=[0 0 0]  TranslationROffset=0  TranslationROffsetUnits=m  TranslationZOffset=0  TranslationZOffsetUnits=m  TranslationThetaOffset=0  TranslationThetaOffsetUnits=deg  RotationMethod=StandardAxis  RotationAngleUnits=deg  RotationStandardAxis=+Z  RotationAngle=180  RotationArbitraryAxis=[0 0 1]  FollAlignAxisA=+X  BaseAlignAxisA=+Y  FollAlignAxisB=+Y  BaseAlignAxisB=+Z  RotationMatrix=[1 0 0; 0 1 0; 0 0 1]  BlockFunction=simmechanics.library.frames_transforms.rigid_transform
  Transform G Arc3 : sm_lib/Frames and Transforms/Rigid Transform  TranslationMethod=StandardAxis  TranslationLengthUnit=m  TranslationStandardAxis=-Y  TranslationStandardOffset=d_genv_ctr_to_xcir  TranslationCartesianOffset=[0 0 0]  TranslationROffset=0  TranslationROffsetUnits=m  TranslationZOffset=0  TranslationZOffsetUnits=m  TranslationThetaOffset=0  TranslationThetaOffsetUnits=deg  RotationMethod=StandardAxis  RotationAngleUnits=deg  RotationStandardAxis=+Z  RotationAngle=90  RotationArbitraryAxis=[0 0 1]  FollAlignAxisA=+X  BaseAlignAxisA=+Y  FollAlignAxisB=+Y  BaseAlignAxisB=+Z  RotationMatrix=[1 0 0; 0 1 0; 0 0 1]  BlockFunction=simmechanics.library.frames_transforms.rigid_transform
  Transform G Arc4 : sm_lib/Frames and Transforms/Rigid Transform  TranslationMethod=StandardAxis  TranslationLengthUnit=m  TranslationStandardAxis=-X  TranslationStandardOffset=d_genv_ctr_to_xcir  TranslationCartesianOffset=[0 0 0]  TranslationROffset=0  TranslationROffsetUnits=m  TranslationZOffset=0  TranslationZOffsetUnits=m  TranslationThetaOffset=0  TranslationThetaOffsetUnits=deg  RotationMethod=StandardAxis  RotationAngleUnits=deg  RotationStandardAxis=+Z  RotationAngle=0  RotationArbitraryAxis=[0 0 1]  FollAlignAxisA=+X  BaseAlignAxisA=+Y  FollAlignAxisB=+Y  BaseAlignAxisB=+Z  RotationMatrix=[1 0 0; 0 1 0; 0 0 1]  BlockFunction=simmechanics.library.frames_transforms.rigid_transform
  Transform Ref DShl : sm_lib/Frames and Transforms/Rigid Transform  TranslationMethod=StandardAxis  TranslationLengthUnit=m  TranslationStandardAxis=+X  TranslationStandardOffset=r_genv_xcir  TranslationCartesianOffset=[0 0 0]  TranslationROffset=0  TranslationROffsetUnits=m  TranslationZOffset=0  TranslationZOffsetUnits=m  TranslationThetaOffset=0  TranslationThetaOffsetUnits=deg  RotationMethod=None  RotationAngleUnits=deg  RotationStandardAxis=+Z  RotationAngle=0  RotationArbitraryAxis=[0 0 1]  FollAlignAxisA=+X  BaseAlignAxisA=+Y  FollAlignAxisB=+Y  BaseAlignAxisB=+Z  RotationMatrix=[1 0 0; 0 1 0; 0 0 1]  BlockFunction=simmechanics.library.frames_transforms.rigid_transform
  Transform p1 cir : sm_lib/Frames and Transforms/Rigid Transform  TranslationMethod=StandardAxis  TranslationLengthUnit=m  TranslationStandardAxis=+X  TranslationStandardOffset=r_shld_cir  TranslationCartesianOffset=[0 0 0]  TranslationROffset=0  TranslationROffsetUnits=m  TranslationZOffset=0  TranslationZOffsetUnits=m  TranslationThetaOffset=0  TranslationThetaOffsetUnits=deg  RotationMethod=None  RotationAngleUnits=deg  RotationStandardAxis=+Z  RotationAngle=0  RotationArbitraryAxis=[0 0 1]  FollAlignAxisA=+X  BaseAlignAxisA=+Y  FollAlignAxisB=+Y  BaseAlignAxisB=+Z  RotationMatrix=[1 0 0; 0 1 0; 0 0 1]  BlockFunction=simmechanics.library.frames_transforms.rigid_transform
  RinB : PMIOPort  Port=1  Side=Left
  CirF : PMIOPort  Port=2  Side=Right
  wires:
  Circle to Ring Arc1 SpB/1 -> Sensing7/1(S)
  "Circle to Ring Arc1 SpA "/1 -> Sensing6/1(S)
  Circle to Ring Arc4 SpB/1 -> Sensing5/1(S)
  Circle to Ring Arc4 SpA/1 -> Sensing4/1(S)
  Circle to Ring Arc3 SpB/1 -> Sensing3/1(S)
  Circle to Ring Arc3 SpA/1 -> Sensing2/1(S)
  Circle to Ring Arc2 SpB/1 -> Sensing1/1(S)
  Circle to Ring Arc2 SpA/1 -> Sensing/1(S)
  Sensing8/1(S) -> Force DShl/1
  connections:
  Circle to Ring Arc3 SpA/RConn1 -- Circle to Ring Arc3 SpB/RConn1 -- Transform G Arc3/RConn1
  Transform Dctr Shl pB/RConn1 -- Circle to Ring Arc3 SpB/LConn1 -- Circle to Ring Arc4 SpB/LConn1 -- Circle to Ring Arc2 SpB/LConn1 -- Circle to Ring Arc1 SpB/LConn1
  Circle to Ring Arc4 SpA/RConn1 -- Circle to Ring Arc4 SpB/RConn1 -- Transform G Arc4/RConn1
  Circle to Ring Arc2 SpA/RConn1 -- Circle to Ring Arc2 SpB/RConn1 -- Transform G Arc2/RConn1
  Transform Dctr Shl pA/RConn1 -- Circle to Ring Arc3 SpA/LConn1 -- Circle to Ring Arc4 SpA/LConn1 -- Circle to Ring Arc2 SpA/LConn1 -- "Circle to Ring Arc1 SpA "/LConn1 -- Transform p1 cir/LConn1
  Transform G Arc1/RConn1 -- "Circle to Ring Arc1 SpA "/RConn1 -- Circle to Ring Arc1 SpB/RConn1 -- Transform Ref DShl/LConn1
  RinB/RConn1 -- Transform G Arc3/LConn1 -- Transform G Arc4/LConn1 -- Transform G Arc2/LConn1 -- Transform G Arc1/LConn1
  CirF/RConn1 -- Transform Dctr Shl pA/LConn1 -- Transform Dctr Shl pB/LConn1

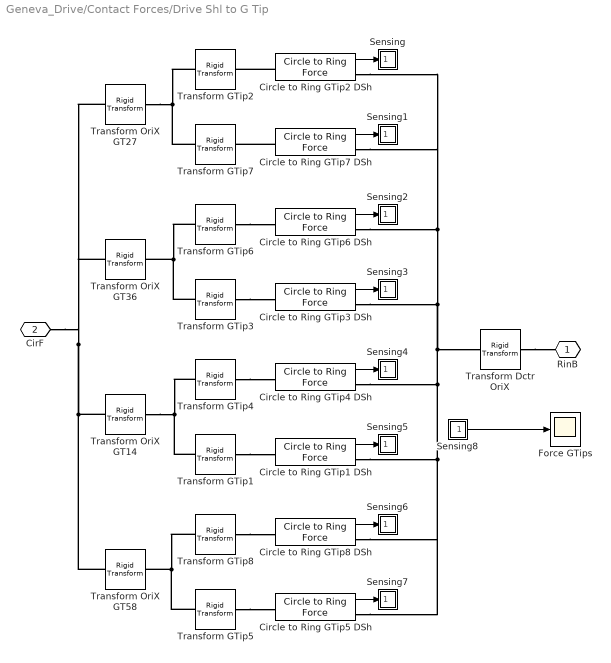
== system Geneva_Drive/Contact Forces/Drive Shl to G Tip ==
  Circle to Ring GTip1 DSh : Contact_Forces_Lib/2D/Circle to Ring Force  radius_circle=r_genv_cir  radius_ring=r_shld-d_shld/2  d_ring=d_shld  active_angle=[-90 180]  force_law=Linear  k_contact=k_contact  b_contact=b_contact  pen_full_damp_F=1e-4  pen_exponent=1  custom_param_1=1  custom_param_2=1  friction_law=None  mu_kinetic=0.5  mu_static=0.7  v_thr=0.001
  Circle to Ring GTip2 DSh : Contact_Forces_Lib/2D/Circle to Ring Force  radius_circle=r_genv_cir  radius_ring=r_shld-d_shld/2  d_ring=d_shld  active_angle=[-90 180]  force_law=Linear  k_contact=k_contact  b_contact=b_contact  pen_full_damp_F=1e-4  pen_exponent=1  custom_param_1=1  custom_param_2=1  friction_law=None  mu_kinetic=0.5  mu_static=0.7  v_thr=0.001
  Circle to Ring GTip3 DSh : Contact_Forces_Lib/2D/Circle to Ring Force  radius_circle=r_genv_cir  radius_ring=r_shld-d_shld/2  d_ring=d_shld  active_angle=[-90 180]  force_law=Linear  k_contact=k_contact  b_contact=b_contact  pen_full_damp_F=1e-4  pen_exponent=1  custom_param_1=1  custom_param_2=1  friction_law=None  mu_kinetic=0.5  mu_static=0.7  v_thr=0.001
  Circle to Ring GTip4 DSh : Contact_Forces_Lib/2D/Circle to Ring Force  radius_circle=r_genv_cir  radius_ring=r_shld-d_shld/2  d_ring=d_shld  active_angle=[-90 180]  force_law=Linear  k_contact=k_contact  b_contact=b_contact  pen_full_damp_F=1e-4  pen_exponent=1  custom_param_1=1  custom_param_2=1  friction_law=None  mu_kinetic=0.5  mu_static=0.7  v_thr=0.001
  Circle to Ring GTip5 DSh : Contact_Forces_Lib/2D/Circle to Ring Force  radius_circle=r_genv_cir  radius_ring=r_shld-d_shld/2  d_ring=d_shld  active_angle=[-90 180]  force_law=Linear  k_contact=k_contact  b_contact=b_contact  pen_full_damp_F=1e-4  pen_exponent=1  custom_param_1=1  custom_param_2=1  friction_law=None  mu_kinetic=0.5  mu_static=0.7  v_thr=0.001
  Circle to Ring GTip6 DSh : Contact_Forces_Lib/2D/Circle to Ring Force  radius_circle=r_genv_cir  radius_ring=r_shld-d_shld/2  d_ring=d_shld  active_angle=[-90 180]  force_law=Linear  k_contact=k_contact  b_contact=b_contact  pen_full_damp_F=1e-4  pen_exponent=1  custom_param_1=1  custom_param_2=1  friction_law=None  mu_kinetic=0.5  mu_static=0.7  v_thr=0.001
  Circle to Ring GTip7 DSh : Contact_Forces_Lib/2D/Circle to Ring Force  radius_circle=r_genv_cir  radius_ring=r_shld-d_shld/2  d_ring=d_shld  active_angle=[-90 180]  force_law=Linear  k_contact=k_contact  b_contact=b_contact  pen_full_damp_F=1e-4  pen_exponent=1  custom_param_1=1  custom_param_2=1  friction_law=None  mu_kinetic=0.5  mu_static=0.7  v_thr=0.001
  Circle to Ring GTip8 DSh : Contact_Forces_Lib/2D/Circle to Ring Force  radius_circle=r_genv_cir  radius_ring=r_shld-d_shld/2  d_ring=d_shld  active_angle=[-90 180]  force_law=Linear  k_contact=k_contact  b_contact=b_contact  pen_full_damp_F=1e-4  pen_exponent=1  custom_param_1=1  custom_param_2=1  friction_law=None  mu_kinetic=0.5  mu_static=0.7  v_thr=0.001
  Force GTips : Scope
      settings: TimeRange=30  YMin=0  YMax=0.9  SaveName=ScopeData2
  Sensing : Subsystem
  Sensing1 : Subsystem
  Sensing2 : Subsystem
  Sensing3 : Subsystem
  Sensing4 : Subsystem
  Sensing5 : Subsystem
  Sensing6 : Subsystem
  Sensing7 : Subsystem
  Sensing8 : Subsystem
  Transform Dctr OriX : sm_lib/Frames and Transforms/Rigid Transform  TranslationMethod=None  TranslationLengthUnit=m  TranslationStandardAxis=+Z  TranslationStandardOffset=0  TranslationCartesianOffset=[0 0 0]  TranslationROffset=0  TranslationROffsetUnits=m  TranslationZOffset=0  TranslationZOffsetUnits=m  TranslationThetaOffset=0  TranslationThetaOffsetUnits=deg  RotationMethod=AlignedAxes  RotationAngleUnits=deg  RotationStandardAxis=+Z  RotationAngle=180  RotationArbitraryAxis=[0 0 1]  FollAlignAxisA=+X  BaseAlignAxisA=-X  FollAlignAxisB=+Z  BaseAlignAxisB=-Z  RotationMatrix=[1 0 0; 0 1 0; 0 0 1]  BlockFunction=simmechanics.library.frames_transforms.rigid_transform
  Transform GTip{1,3,5,7} (4 alike) : sm_lib/Frames and Transforms/Rigid Transform  TranslationMethod=Cartesian  TranslationLengthUnit=m  TranslationStandardAxis=+Y  TranslationStandardOffset=0.1405  TranslationCartesianOffset=[-0.022 -0.139 0]  TranslationROffset=0  TranslationROffsetUnits=m  TranslationZOffset=0  TranslationZOffsetUnits=m  TranslationThetaOffset=0  TranslationThetaOffsetUnits=deg  RotationMethod=None  RotationAngleUnits=deg  RotationStandardAxis=+Z  RotationAngle=45  RotationArbitraryAxis=[0 0 1]  FollAlignAxisA=+X  BaseAlignAxisA=+Y  FollAlignAxisB=+Y  BaseAlignAxisB=+Z  RotationMatrix=[1 0 0; 0 1 0; 0 0 1]  BlockFunction=simmechanics.library.frames_transforms.rigid_transform
  Transform GTip{2,4,6,8} (4 alike) : sm_lib/Frames and Transforms/Rigid Transform  TranslationMethod=Cartesian  TranslationLengthUnit=m  TranslationStandardAxis=+Y  TranslationStandardOffset=0.1405  TranslationCartesianOffset=[-0.022 0.139 0]  TranslationROffset=0  TranslationROffsetUnits=m  TranslationZOffset=0  TranslationZOffsetUnits=m  TranslationThetaOffset=0  TranslationThetaOffsetUnits=deg  RotationMethod=None  RotationAngleUnits=deg  RotationStandardAxis=+Z  RotationAngle=45  RotationArbitraryAxis=[0 0 1]  FollAlignAxisA=+X  BaseAlignAxisA=+Y  FollAlignAxisB=+Y  BaseAlignAxisB=+Z  RotationMatrix=[1 0 0; 0 1 0; 0 0 1]  BlockFunction=simmechanics.library.frames_transforms.rigid_transform
  Transform OriX GT14 : sm_lib/Frames and Transforms/Rigid Transform  TranslationMethod=None  TranslationLengthUnit=m  TranslationStandardAxis=+Z  TranslationStandardOffset=0  TranslationCartesianOffset=[0 0 0]  TranslationROffset=0  TranslationROffsetUnits=m  TranslationZOffset=0  TranslationZOffsetUnits=m  TranslationThetaOffset=0  TranslationThetaOffsetUnits=deg  RotationMethod=StandardAxis  RotationAngleUnits=deg  RotationStandardAxis=+Z  RotationAngle=225  RotationArbitraryAxis=[0 0 1]  FollAlignAxisA=+X  BaseAlignAxisA=+Y  FollAlignAxisB=+Y  BaseAlignAxisB=+Z  RotationMatrix=[1 0 0; 0 1 0; 0 0 1]  BlockFunction=simmechanics.library.frames_transforms.rigid_transform
  Transform OriX GT27 : sm_lib/Frames and Transforms/Rigid Transform  TranslationMethod=None  TranslationLengthUnit=m  TranslationStandardAxis=+Z  TranslationStandardOffset=0  TranslationCartesianOffset=[0 0 0]  TranslationROffset=0  TranslationROffsetUnits=m  TranslationZOffset=0  TranslationZOffsetUnits=m  TranslationThetaOffset=0  TranslationThetaOffsetUnits=deg  RotationMethod=StandardAxis  RotationAngleUnits=deg  RotationStandardAxis=+Z  RotationAngle=315  RotationArbitraryAxis=[0 0 1]  FollAlignAxisA=+X  BaseAlignAxisA=+Y  FollAlignAxisB=+Y  BaseAlignAxisB=+Z  RotationMatrix=[1 0 0; 0 1 0; 0 0 1]  BlockFunction=simmechanics.library.frames_transforms.rigid_transform
  Transform OriX GT36 : sm_lib/Frames and Transforms/Rigid Transform  TranslationMethod=None  TranslationLengthUnit=m  TranslationStandardAxis=+Z  TranslationStandardOffset=0  TranslationCartesianOffset=[0 0 0]  TranslationROffset=0  TranslationROffsetUnits=m  TranslationZOffset=0  TranslationZOffsetUnits=m  TranslationThetaOffset=0  TranslationThetaOffsetUnits=deg  RotationMethod=StandardAxis  RotationAngleUnits=deg  RotationStandardAxis=+Z  RotationAngle=135  RotationArbitraryAxis=[0 0 1]  FollAlignAxisA=+X  BaseAlignAxisA=+Y  FollAlignAxisB=+Y  BaseAlignAxisB=+Z  RotationMatrix=[1 0 0; 0 1 0; 0 0 1]  BlockFunction=simmechanics.library.frames_transforms.rigid_transform
  Transform OriX GT58 : sm_lib/Frames and Transforms/Rigid Transform  TranslationMethod=None  TranslationLengthUnit=m  TranslationStandardAxis=+Z  TranslationStandardOffset=0  TranslationCartesianOffset=[0 0 0]  TranslationROffset=0  TranslationROffsetUnits=m  TranslationZOffset=0  TranslationZOffsetUnits=m  TranslationThetaOffset=0  TranslationThetaOffsetUnits=deg  RotationMethod=StandardAxis  RotationAngleUnits=deg  RotationStandardAxis=+Z  RotationAngle=45  RotationArbitraryAxis=[0 0 1]  FollAlignAxisA=+X  BaseAlignAxisA=+Y  FollAlignAxisB=+Y  BaseAlignAxisB=+Z  RotationMatrix=[1 0 0; 0 1 0; 0 0 1]  BlockFunction=simmechanics.library.frames_transforms.rigid_transform
  RinB : PMIOPort  Port=1  Side=Right
  CirF : PMIOPort  Port=2  Side=Left
  wires:
  Sensing8/1(S) -> Force GTips/1
  Circle to Ring GTip5 DSh/1 -> Sensing7/1(S)
  Circle to Ring GTip8 DSh/1 -> Sensing6/1(S)
  Circle to Ring GTip2 DSh/1 -> Sensing/1(S)
  Circle to Ring GTip6 DSh/1 -> Sensing2/1(S)
  Circle to Ring GTip4 DSh/1 -> Sensing4/1(S)
  Circle to Ring GTip7 DSh/1 -> Sensing1/1(S)
  Circle to Ring GTip3 DSh/1 -> Sensing3/1(S)
  Circle to Ring GTip1 DSh/1 -> Sensing5/1(S)
  connections:
  Transform GTip8/LConn1 -- Transform GTip5/LConn1 -- Transform OriX GT58/RConn1
  Transform GTip5/RConn1 -- Circle to Ring GTip5 DSh/LConn1
  Circle to Ring GTip3 DSh/RConn1 -- Transform Dctr OriX/RConn1 -- Circle to Ring GTip4 DSh/RConn1 -- Circle to Ring GTip1 DSh/RConn1 -- Circle to Ring GTip8 DSh/RConn1 -- Circle to Ring GTip5 DSh/RConn1 -- Circle to Ring GTip7 DSh/RConn1 -- Circle to Ring GTip2 DSh/RConn1 -- Circle to Ring GTip6 DSh/RConn1
  Transform GTip6/RConn1 -- Circle to Ring GTip6 DSh/LConn1
  Circle to Ring GTip7 DSh/LConn1 -- Transform GTip7/RConn1
  Circle to Ring GTip2 DSh/LConn1 -- Transform GTip2/RConn1
  Transform GTip8/RConn1 -- Circle to Ring GTip8 DSh/LConn1
  Transform GTip1/RConn1 -- Circle to Ring GTip1 DSh/LConn1
  Transform GTip4/RConn1 -- Circle to Ring GTip4 DSh/LConn1
  Transform GTip3/RConn1 -- Circle to Ring GTip3 DSh/LConn1
  Transform OriX GT27/RConn1 -- Transform GTip2/LConn1 -- Transform GTip7/LConn1
  Transform GTip3/LConn1 -- Transform GTip6/LConn1 -- Transform OriX GT36/RConn1
  Transform OriX GT14/LConn1 -- Transform OriX GT58/LConn1 -- Transform OriX GT36/LConn1 -- Transform OriX GT27/LConn1 -- CirF/RConn1
  Transform GTip1/LConn1 -- Transform GTip4/LConn1 -- Transform OriX GT14/RConn1
  Transform Dctr OriX/LConn1 -- RinB/RConn1

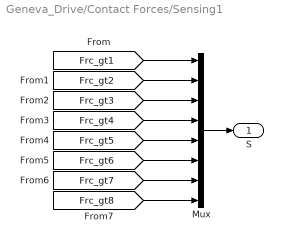
== system Geneva_Drive/Contact Forces/Sensing1 ==
  Mux : Mux  Inputs=8
  S : Outport
  wires:
  [Frc_gt6] -> Mux/6
  [Frc_gt5] -> Mux/5
  [Frc_gt8] -> Mux/8
  [Frc_gt7] -> Mux/7
  [Frc_gt4] -> Mux/4
  [Frc_gt2] -> Mux/2
  [Frc_gt3] -> Mux/3
  [Frc_gt1] -> Mux/1
  Mux/1 -> S/1

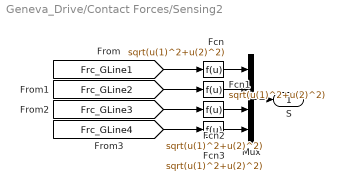
== system Geneva_Drive/Contact Forces/Sensing2 ==
  Fcn{,1..3} (4 alike) : Fcn  Expr=sqrt(u(1)^2+u(2)^2)
  Mux : Mux
  S : Outport
  wires:
  Fcn3/1 -> Mux/4
  Fcn2/1 -> Mux/3
  Fcn1/1 -> Mux/2
  Fcn/1 -> Mux/1
  [Frc_GLine4] -> Fcn3/1
  [Frc_GLine2] -> Fcn1/1
  [Frc_GLine3] -> Fcn2/1
  [Frc_GLine1] -> Fcn/1
  Mux/1 -> S/1

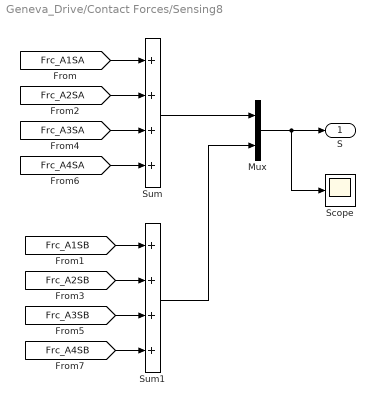
== system Geneva_Drive/Contact Forces/Sensing8 ==
  Mux : Mux  Inputs=2
  Scope : Scope
      settings: TimeRange=30  YMin=-0.4  YMax=0  SaveName=ScopeData6
  Sum : Sum  Inputs=++++
  Sum1 : Sum  Inputs=++++
  S : Outport
  wires:
  Sum1/1 -> Mux/2
  Sum/1 -> Mux/1
  [Frc_A3SB] -> Sum1/3
  [Frc_A2SB] -> Sum1/2
  [Frc_A4SB] -> Sum1/4
  [Frc_A1SB] -> Sum1/1
  [Frc_A1SA] -> Sum/1
  [Frc_A4SA] -> Sum/4
  [Frc_A2SA] -> Sum/2
  [Frc_A3SA] -> Sum/3
  Mux/1 -> S/1, Scope/1
